simulink model "DiscretePID"  (R2020a)
settings: Solver=VariableStepAuto  StartTime=0.0  StopTime=10  RelTol=1e-3
values from neighbouring files (symbols this model uses):
  Kd = -0.00042527    [C.mat]    (also in updateParameters.m = 0)
  Ki = 0.5044    [C.mat]    (also in updateParameters.m = 1.6452)
  Kp = 0.058    [C.mat]    (also in updateParameters.m = 0.0165)
  N = 22    [C.mat]    (also in updateParameters.m = 100)
  output_limits = [-12 12]    [C.mat]    (also in updateParameters.m)
  sw_b = 0.0411    [C.mat]    (also in updateParameters.m = 1)
  sw_c = 0.2304    [C.mat]    (also in updateParameters.m = 1)
  TFd = [0.02722 1]    [C.mat]    (also in updateParameters.m = [tau 1])
  TFn = 2.305    [C.mat]    (also in updateParameters.m)
  Ts = 0.025    [C.mat]    (also in updateParameters.m = 0.02)
libraries: simulink x1
settings Model: Creator=aaron  LastModifiedBy=aaron

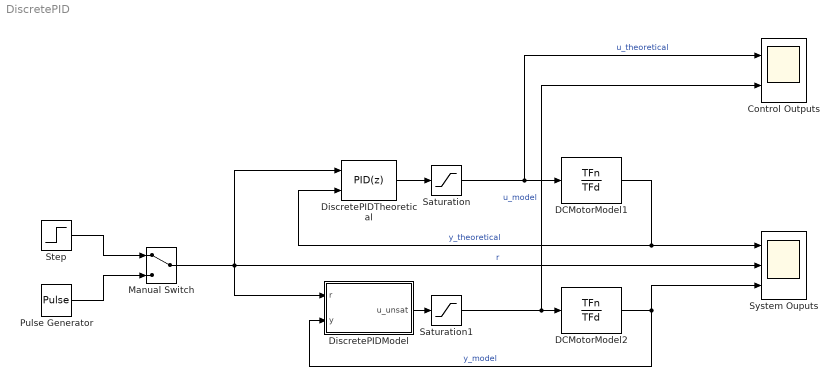
== system DiscretePID ==
  Control Outputs : Scope  NumInputPorts=2
  DCMotorModel1 : TransferFcn  Numerator=TFn  Denominator=TFd
  DCMotorModel2 : TransferFcn  Numerator=TFn  Denominator=TFd
  DiscretePIDModel : Subsystem
  DiscretePIDTheoretical : simulink/Continuous/PID Controller (2DOF)  Controller=PID  Form=Parallel  TimeDomain=Discrete-time  UseExternalTs=off  SampleTime=Ts  IntegratorMethod=Forward Euler  FilterMethod=Backward Euler  ControllerParametersSource=internal  P=Kp  I=Ki  D=Kd  UseFilter=on  N=N  b=sw_b  c=sw_c  TunerSelectOption=Transfer Function Based (PID Tuner App)  InitialConditionSource=internal  InitialConditionForIntegrator=0  InitialConditionForFilter=0  DifferentiatorICPrevScaledInput=0  ExternalReset=none  TrackingMode=off  Kt=1  LimitOutput=off  UpperSaturationLimit=output_limits(2)  LowerSaturationLimit=output_limits(1)  LinearizeAsGain=off  AntiWindupMode=none  Kb=1  POutMin=[]  POutMax=[]  IOutMin=[]  IOutMax=[]  DOutMin=[]  DOutMax=[]  NOutMin=[]  NOutMax=[]  bOutMin=[]  bOutMax=[]  cOutMin=[]  cOutMax=[]  SumOutMin=[]  SumOutMax=[]  SaturationOutMin=[]  SaturationOutMax=[]  PParamMin=[]  PParamMax=[]  IParamMin=[]  IParamMax=[]  DParamMin=[]  DParamMax=[]  NParamMin=[]  NParamMax=[]  bParamMin=[]  bParamMax=[]  cParamMin=[]  cParamMax=[]  KbParamMin=[]  KbParamMax=[]  KtParamMin=[]  KtParamMax=[]  KbOutMin=[]  KbOutMax=[]  KtOutMin=[]  KtOutMax=[]  IntegratorOutMin=[]  IntegratorOutMax=[]  FilterOutMin=[]  FilterOutMax=[]  SumI1OutMin=[]  SumI1OutMax=[]  SumI2OutMin=[]  SumI2OutMax=[]  SumI3OutMin=[]  SumI3OutMax=[]  SumI4OutMin=[]  SumI4OutMax=[]  SumDOutMin=[]  SumDOutMax=[]  Sum1OutMin=[]  Sum1OutMax=[]  Sum2OutMin=[]  Sum2OutMax=[]  Sum3OutMin=[]  Sum3OutMax=[]  DifferentiatorOutMin=[]  DifferentiatorOutMax=[]  FilterDiffOutCoefMin=[]  FilterDiffOutCoefMax=[]  ReciprocalOutMin=[]  ReciprocalOutMax=[]  SumDenOutMin=[]  SumDenOutMax=[]  SumNumOutMin=[]  SumNumOutMax=[]  DivideOutMin=[]  DivideOutMax=[]  UdiffTsProdOutMin=[]  UdiffTsProdOutMax=[]  NTsProdOutMin=[]  NTsProdOutMax=[]  UintegralTsProdOutMin=[]  UintegralTsProdOutMax=[]  UngainTsProdOutMin=[]  UngainTsProdOutMax=[]  IntegratorContinuousStateAttributes=''  IntegratorStateMustResolveToSignalObject=off  IntegratorRTWStateStorageClass=Auto  FilterContinuousStateAttributes=''  FilterStateMustResolveToSignalObject=off  FilterRTWStateStorageClass=Auto  ParallelPVariant=InternalParameters  IdealPVariant=Disabled  IVariant=InternalParameters  DVariant=InternalParameters  bVariant=InternalParameters  cVariant=InternalParameters  IntegratorVariant=Discrete  SatVariant=Disabled  AWVariant=Passthrough  PCopyVariant=Disabled  TRVariant=Disabled  FdbkBlocksVariant=Forward  IdealPFdbkVariant=Disabled  SatFdbkVariant=Disabled  DerivativeFilterVariant=BackwardEulerFilter  NVariant=InternalParameters  NCopyVariant=InternalParameters  FilterICVariant=InternalICsFilter  IntegratorICVariant=InternalICs  ExternalResetVariant=Disabled  TRSumVariant=Passthrough  SumFdbkVariant=Disabled  SumVariant=Sum_PID  TsampFilterVariant=InternalTs  TsampNgainVariant=Passthrough  TsampIntegralVariant=Passthrough
  Manual Switch : ManualSwitch
  Pulse Generator : DiscretePulseGenerator  PulseType=Time based  Period=4  PulseWidth=50
  Saturation : Saturate  UpperLimit=output_limits(2)  LowerLimit=output_limits(1)
  Saturation1 : Saturate  UpperLimit=output_limits(2)  LowerLimit=output_limits(1)
  Step : Step  Time=5  Before=10  After=20  SampleTime=Ts
  System Ouputs : Scope  NumInputPorts=3
  wires:
  Manual Switch/1 -> DiscretePIDModel/1(r), DiscretePIDTheoretical/1, System Ouputs/2  "r"
  DCMotorModel1/1 -> System Ouputs/1, DiscretePIDTheoretical/2  "y_theoretical"
  DiscretePIDTheoretical/1 -> Saturation/1
  DCMotorModel2/1 -> System Ouputs/3, DiscretePIDModel/2(y)  "y_model"
  Pulse Generator/1 -> Manual Switch/2
  Step/1 -> Manual Switch/1
  Saturation/1 -> DCMotorModel1/1, Control Outputs/1  "u_theoretical"
  Saturation1/1 -> Control Outputs/2, DCMotorModel2/1  "u_model"
  DiscretePIDModel/1(u_unsat) -> Saturation1/1

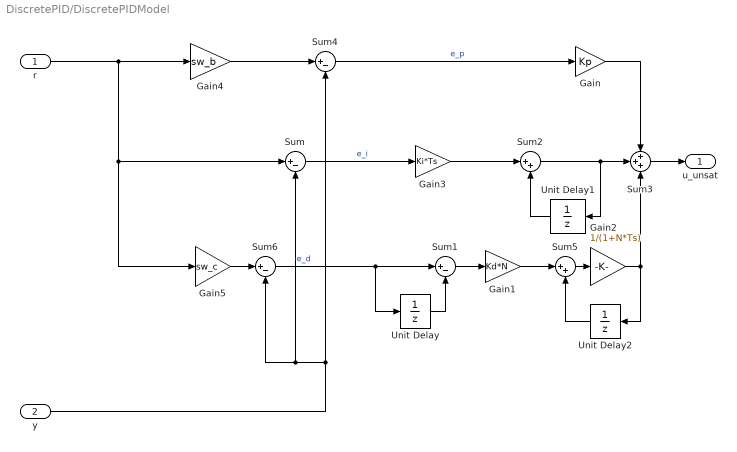
== system DiscretePID/DiscretePIDModel ==
  r : Inport
  y : Inport  Port=2
  Gain : Gain  Gain=Kp  OutDataTypeStr=Inherit: Same as input
  Gain1 : Gain  Gain=Kd*N  OutDataTypeStr=Inherit: Same as input
  Gain2 : Gain  Gain=1/(1+N*Ts)  OutDataTypeStr=Inherit: Same as input
  Gain3 : Gain  Gain=Ki*Ts  OutDataTypeStr=Inherit: Same as input
  Gain4 : Gain  Gain=sw_b
  Gain5 : Gain  Gain=sw_c
  Sum : Sum  Inputs=|+-  OutDataTypeStr=double
  Sum1 : Sum  Inputs=|+-  AccumDataTypeStr=double  OutDataTypeStr=double
  Sum2 : Sum  Inputs=|++  OutDataTypeStr=Inherit: Same as first input
  Sum3 : Sum  Inputs=+++  OutMin=output_limits(1)  OutMax=output_limits(2)  OutDataTypeStr=double
  Sum4 : Sum  Inputs=|+-
  Sum5 : Sum  Inputs=|++  OutDataTypeStr=Inherit: Same as first input
  Sum6 : Sum  Inputs=|+-  OutDataTypeStr=double
  Unit Delay : UnitDelay  SampleTime=Ts  HasFrameUpgradeWarning=on
  Unit Delay1 : UnitDelay  SampleTime=Ts  HasFrameUpgradeWarning=on
  Unit Delay2 : UnitDelay  SampleTime=Ts  HasFrameUpgradeWarning=on
  u_unsat : Outport
  wires:
  Gain3/1 -> Sum2/1
  Gain5/1 -> Sum6/1
  Sum4/1 -> Gain/1  "e_p"
  Sum2/1 -> Unit Delay1/1, Sum3/2
  Unit Delay2/1 -> Sum5/2
  r/1 -> Gain5/1, Sum/1, Gain4/1
  Sum1/1 -> Gain1/1
  Sum3/1 -> u_unsat/1
  Sum5/1 -> Gain2/1
  y/1 -> Sum4/2, Sum/2, Sum6/2
  Gain1/1 -> Sum5/1
  Gain4/1 -> Sum4/1
  Sum/1 -> Gain3/1  "e_i"
  Sum6/1 -> Unit Delay/1, Sum1/1  "e_d"
  Unit Delay/1 -> Sum1/2
  Gain2/1 -> Unit Delay2/1, Sum3/3
  Gain/1 -> Sum3/1
  Unit Delay1/1 -> Sum2/2
